simulink model "Power_Model_Official_Pars"  (R2023a)
settings: Solver=ode23t  StartTime=0.0  StopTime=1000  FixedStep=0.01  MaxStep=0.01  RelTol=1e-3  AbsTol=1e-3
values from neighbouring files (symbols this model uses):
  anode_tube_D = 0.01    [fuel_cell_battery_par.mat]
  cathode_tube_D = 0.05    [fuel_cell_battery_par.mat]
  comp_rpm_TLU = [0 1800 3600]    [fuel_cell_battery_par.mat]
  coolant_num_layers = 20    [fuel_cell_battery_par.mat]
  coolant_num_passes = 12    [fuel_cell_battery_par.mat]
  coolant_tube_D = 0.05    [fuel_cell_battery_par.mat]
  coolant_w_channels = 1    [fuel_cell_battery_par.mat]
  env_p = 0.101325    [fuel_cell_battery_par.mat]
  env_T = 20    [fuel_cell_battery_par.mat]
  env_yH20 = 0.0115436377169    [fuel_cell_battery_par.mat]
  env_yO2 = 0.21    [fuel_cell_battery_par.mat]
  radiator_air_area_fins = 11.5625    [fuel_cell_battery_par.mat]
  radiator_air_area_primary = 1.223125    [fuel_cell_battery_par.mat]
  radiator_eta_fin = 0.7    [fuel_cell_battery_par.mat]
  radiator_N_tubes = 25    [fuel_cell_battery_par.mat]
  radiator_rho = 2700    [fuel_cell_battery_par.mat]
  radiator_t_wall = 0.0001    [fuel_cell_battery_par.mat]
  radiator_tube_H = 0.0015    [fuel_cell_battery_par.mat]
  radiator_W = 0.025    [fuel_cell_battery_par.mat]
  stack_area = 280    [fuel_cell_battery_par.mat]
  stack_iL = 1.4    [fuel_cell_battery_par.mat]
  stack_mea_rho = 1800    [fuel_cell_battery_par.mat]
  stack_num_cells = 400    [fuel_cell_battery_par.mat]
  stack_num_channels = 8    [fuel_cell_battery_par.mat]
  stack_t_gdl = 250    [fuel_cell_battery_par.mat]
  stack_t_membrane = 125    [fuel_cell_battery_par.mat]
  stack_w_channels = 1    [fuel_cell_battery_par.mat]
undefined symbols (not defined in the file or in its folder): Bat, f_fc_auxpower, f_fc_currcmd_bpt, f_fc_h2flow, f_fc_heatflow, f_fc_tmpcmd_bpt, f_fc_voltage, Mot, N2_T
libraries: fl_lib x170, nesl_utility x78, FuelCell_lib x32, simulink x5, slpidlib x4, ee_lib x3, autolibshared x1, batteryecm_lib x1, simulink_extras x1
(part 5 of 9)

== system Power_Model_Official_Pars/氧气供给(压缩机)/压缩机查表 ==
  note: 转速_压力比_流量
  Absolute Reference (MA) : fl_lib/Moist Air/Elements/Absolute Reference (MA)
  Absolute Reference (MA)1 : fl_lib/Moist Air/Elements/Absolute Reference (MA)
  Corrected Flow Table : fl_lib/Physical Signals/Lookup Tables/PS Lookup Table (2D)  x1=comp_p_ratio_TLU Pa/Pa  x2=comp_rpm_TLU rpm  f=comp_mdot_corr_TLU kg/s  interp_method=simscape.enum.interpolation.linear  extrap_method=simscape.enum.extrapolation.nearest
  PS Divide : fl_lib/Physical Signals/Functions/PS Divide
  Pressure & Temperature Sensor (MA) : fl_lib/Moist Air/Sensors/Pressure & Temperature Sensor (MA)  reference=foundation.enum.MeasurementReference.difference  pressure=true  pressure_spec=foundation.enum.PressureMeasementSpec.Absolute  temperature=true
      settings: InternalSimscapePortConfiguration="{\"Bottom\":[{\"id\":\"T\",\"label\":\"T\",\"type\":\"output\"}],\"Left\":[{\"id\":\"A\",\"label\":\"A\",\"type\":\"foundation.moist_air.moist_air\"}],\"Right\":[{\"id\":\"B\",\"label\":\"B\",\"type\":\"foundation.moist_air.moist_air\"},{\"id\":\"P\",\"label\":\"P\",\"type\":\"output\"}],\"Top\":[]}"
  Pressure & Temperature Sensor (MA)1 : fl_lib/Moist Air/Sensors/Pressure & Temperature Sensor (MA)  reference=foundation.enum.MeasurementReference.difference  pressure=true  pressure_spec=foundation.enum.PressureMeasementSpec.Absolute  temperature=true
      settings: InternalSimscapePortConfiguration="{\"Bottom\":[{\"id\":\"T\",\"label\":\"T\",\"type\":\"output\"}],\"Left\":[{\"id\":\"A\",\"label\":\"A\",\"type\":\"foundation.moist_air.moist_air\"}],\"Right\":[{\"id\":\"B\",\"label\":\"B\",\"type\":\"foundation.moist_air.moist_air\"},{\"id\":\"P\",\"label\":\"P\",\"type\":\"output\"}],\"Top\":[]}"
  mdot : PMIOPort  Side=Left
  in : PMIOPort  Port=2  Side=Right
  rpm : PMIOPort  Port=3  Side=Right
  out : PMIOPort  Port=4  Side=Right
  connections:
  Pressure & Temperature Sensor (MA)1/RConn2 -- PS Divide/LConn1
  Absolute Reference (MA)1/LConn1 -- Pressure & Temperature Sensor (MA)1/RConn1
  PS Divide/RConn1 -- Corrected Flow Table/LConn1
  rpm/RConn1 -- Corrected Flow Table/LConn2
  Pressure & Temperature Sensor (MA)/RConn2 -- PS Divide/LConn2
  in/RConn1 -- Pressure & Temperature Sensor (MA)/LConn1
  Absolute Reference (MA)/LConn1 -- Pressure & Temperature Sensor (MA)/RConn1
  Pressure & Temperature Sensor (MA)1/LConn1 -- out/RConn1
  mdot/RConn1 -- Corrected Flow Table/RConn1

== system Power_Model_Official_Pars/阳极加湿器/Proportional Control ==
  RH_set : Inport
  RH_meas : Inport  Port=2
  Gain : Gain  Gain=0.1
  Saturation : Saturate  UpperLimit=inf  LowerLimit=0  ZeroCross=off
  Sum : Sum  Inputs=|+-
  Transfer Fcn : TransferFcn  Denominator=[1 1]
  Mw : Outport
  wires:
  Transfer Fcn/1 -> Mw/1
  Gain/1 -> Saturation/1
  Sum/1 -> Gain/1
  RH_set/1 -> Sum/1
  RH_meas/1 -> Sum/2
  Saturation/1 -> Transfer Fcn/1

== system Power_Model_Official_Pars/阴极加湿器/Proportional Control ==
  RH_set : Inport
  RH_meas : Inport  Port=2
  Gain : Gain  Gain=0.1
  Saturation : Saturate  UpperLimit=inf  LowerLimit=0  ZeroCross=off
  Sum : Sum  Inputs=|+-
  Transfer Fcn : TransferFcn  Denominator=[1 1]
  Mw : Outport
  wires:
  RH_set/1 -> Sum/1
  Sum/1 -> Gain/1
  RH_meas/1 -> Sum/2
  Transfer Fcn/1 -> Mw/1
  Gain/1 -> Saturation/1
  Saturation/1 -> Transfer Fcn/1

== system Power_Model_Official_Pars/阴极排放/Pressure Relief Valve ==
  note: 实际输出压力
  note: 设定输出压力
  Absolute Reference (MA) : fl_lib/Moist Air/Elements/Absolute Reference (MA)
  PS Add : fl_lib/Physical Signals/Functions/PS Add
  PS Constant : fl_lib/Physical Signals/Sources/PS Constant  constant=r_min^2
  PS Gain : fl_lib/Physical Signals/Functions/PS Gain  gain=(r_max^2 - r_min^2)/p_range 1/MPa
  PS Gain1 : fl_lib/Physical Signals/Functions/PS Gain  gain=pi*D^2/4 m^2
  PS Subtract : fl_lib/Physical Signals/Functions/PS Subtract
  Pressure & Temperature Sensor (MA) : fl_lib/Moist Air/Sensors/Pressure & Temperature Sensor (MA)  reference=foundation.enum.MeasurementReference.difference  pressure=true  pressure_spec=foundation.enum.PressureMeasementSpec.Absolute  temperature=true
      settings: InternalSimscapePortConfiguration="{\"Bottom\":[{\"id\":\"T\",\"label\":\"T\",\"type\":\"output\"}],\"Left\":[{\"id\":\"A\",\"label\":\"A\",\"type\":\"foundation.moist_air.moist_air\"}],\"Right\":[{\"id\":\"B\",\"label\":\"B\",\"type\":\"foundation.moist_air.moist_air\"},{\"id\":\"P\",\"label\":\"P\",\"type\":\"output\"}],\"Top\":[]}"
  Valve : fl_lib/Moist Air/Elements/Local Restriction (MA)  restriction_type=foundation.enum.restriction_type.variable  restriction_area=0.001 m^2  min_area=pi*(r_min*D)^2/4 m^2  max_area=pi*(r_max*D)^2/4 m^2  area=pi*D^2/4 m^2  Cd=0.64  B_lam=0.999
  A : PMIOPort  Side=Left
  B : PMIOPort  Port=2  Side=Right
  p_set : PMIOPort  Port=3  Side=Left
  connections:
  p_set/RConn1 -- PS Subtract/LConn2
  Pressure & Temperature Sensor (MA)/RConn2 -- PS Subtract/LConn1
  PS Add/LConn2 -- PS Constant/RConn1
  PS Gain/RConn1 -- PS Add/LConn1
  Pressure & Temperature Sensor (MA)/LConn1 -- A/RConn1 -- Valve/LConn1
  Valve/RConn1 -- B/RConn1
  Absolute Reference (MA)/LConn1 -- Pressure & Temperature Sensor (MA)/RConn1
  PS Gain1/RConn1 -- Valve/LConn2
  PS Gain/LConn1 -- PS Subtract/RConn1
  PS Add/RConn1 -- PS Gain1/LConn1

== system Power_Model_Official_Pars/Electrical Load/Inputs/Drive Cycle Power Demand ==
  From Workspace : FromWorkspace  VariableName=[drive_cycle_time, drive_cycle_power]
  PS Divide : fl_lib/Physical Signals/Functions/PS Divide
  PS-Simulink Converter : nesl_utility/PS-Simulink Converter  PhysicalDomain=network_engine_domain  SubClassName=ps_output  LeftPortType=input  RightPortType=output  PseudoPeriodic=off  Frequencies=[]  VectorFormat=1-D array  Unit=V  AffineConversion=off
  PS-Simulink Converter1 : nesl_utility/PS-Simulink Converter  PhysicalDomain=network_engine_domain  SubClassName=ps_output  LeftPortType=input  RightPortType=output  PseudoPeriodic=off  Frequencies=[]  VectorFormat=1-D array  Unit=A  AffineConversion=off
  Simulink-PS Converter : nesl_utility/Simulink-PS Converter  PhysicalDomain=network_engine_domain  SubClassName=ps_input  LeftPortType=input  RightPortType=output  PseudoPeriodic=off  Frequencies=[]  NoiseDistribution=none  NoiseParameters=[]  Unit=kW  AffineConversion=off  FilteringAndDerivatives=provide  SimscapeFilterOrder=1  InputFilterTimeConstant=0.001  UdotUserProvided=0
  i : PMIOPort  Side=Left
  v : PMIOPort  Port=2  Side=Left
  tag scope: i_stack=global, v_stack=global
  wires:
  From Workspace/1 -> Simulink-PS Converter/1
  PS-Simulink Converter/1 -> [v_stack]
  PS-Simulink Converter1/1 -> [i_stack]
  connections:
  PS Divide/LConn1 -- Simulink-PS Converter/RConn1
  i/RConn1 -- PS Divide/RConn1 -- PS-Simulink Converter1/LConn1
  v/RConn1 -- PS-Simulink Converter/LConn1 -- PS Divide/LConn2

== system Power_Model_Official_Pars/Electrical Load/Inputs/Ramp Current Demand ==
  PS-Simulink Converter : nesl_utility/PS-Simulink Converter  PhysicalDomain=network_engine_domain  SubClassName=ps_output  LeftPortType=input  RightPortType=output  PseudoPeriodic=off  Frequencies=[]  VectorFormat=1-D array  Unit=V  AffineConversion=off
  Ramp : simulink/Sources/Ramp  slope=stack_iL * stack_area /1000  start=0  InitialOutput=1e-6 * stack_iL * stack_area
  Simulink-PS Converter : nesl_utility/Simulink-PS Converter  PhysicalDomain=network_engine_domain  SubClassName=ps_input  LeftPortType=input  RightPortType=output  PseudoPeriodic=off  Frequencies=[]  NoiseDistribution=none  NoiseParameters=[]  Unit=A  AffineConversion=off  FilteringAndDerivatives=provide  SimscapeFilterOrder=1  InputFilterTimeConstant=0.001  UdotUserProvided=0
  i : PMIOPort  Side=Left
  v : PMIOPort  Port=2  Side=Left
  tag scope: i_stack=global, v_stack=global
  wires:
  Ramp/1 -> Simulink-PS Converter/1, [i_stack]
  PS-Simulink Converter/1 -> [v_stack]
  connections:
  Simulink-PS Converter/RConn1 -- i/RConn1
  v/RConn1 -- PS-Simulink Converter/LConn1

== system Power_Model_Official_Pars/Electrical Load/Inputs/Step Current Demand ==
  PS-Simulink Converter : nesl_utility/PS-Simulink Converter  PhysicalDomain=network_engine_domain  SubClassName=ps_output  LeftPortType=input  RightPortType=output  PseudoPeriodic=off  Frequencies=[]  VectorFormat=1-D array  Unit=V  AffineConversion=off
  Simulink-PS Converter : nesl_utility/Simulink-PS Converter  PhysicalDomain=network_engine_domain  SubClassName=ps_input  LeftPortType=input  RightPortType=output  PseudoPeriodic=off  Frequencies=[]  NoiseDistribution=none  NoiseParameters=[]  Unit=A  AffineConversion=off  FilteringAndDerivatives=provide  SimscapeFilterOrder=1  InputFilterTimeConstant=0.001  UdotUserProvided=0
  Step : Step  Time=0  Before=1e-6 * stack_iL * stack_area  After=stack_iL * stack_area  SampleTime=0
  i : PMIOPort  Side=Left
  v : PMIOPort  Port=2  Side=Left
  tag scope: i_stack=global, v_stack=global
  wires:
  Step/1 -> [i_stack], Simulink-PS Converter/1
  PS-Simulink Converter/1 -> [v_stack]
  connections:
  Simulink-PS Converter/RConn1 -- i/RConn1
  PS-Simulink Converter/LConn1 -- v/RConn1

== system Power_Model_Official_Pars/Electrical Load1/Inputs/Drive Cycle Power Demand ==
  From Workspace : FromWorkspace  VariableName=[drive_cycle_time, drive_cycle_power]
  PS Divide : fl_lib/Physical Signals/Functions/PS Divide
  PS-Simulink Converter : nesl_utility/PS-Simulink Converter  PhysicalDomain=network_engine_domain  SubClassName=ps_output  LeftPortType=input  RightPortType=output  PseudoPeriodic=off  Frequencies=[]  VectorFormat=1-D array  Unit=V  AffineConversion=off
  PS-Simulink Converter1 : nesl_utility/PS-Simulink Converter  PhysicalDomain=network_engine_domain  SubClassName=ps_output  LeftPortType=input  RightPortType=output  PseudoPeriodic=off  Frequencies=[]  VectorFormat=1-D array  Unit=A  AffineConversion=off
  Simulink-PS Converter : nesl_utility/Simulink-PS Converter  PhysicalDomain=network_engine_domain  SubClassName=ps_input  LeftPortType=input  RightPortType=output  PseudoPeriodic=off  Frequencies=[]  NoiseDistribution=none  NoiseParameters=[]  Unit=kW  AffineConversion=off  FilteringAndDerivatives=provide  SimscapeFilterOrder=1  InputFilterTimeConstant=0.001  UdotUserProvided=0
  i : PMIOPort  Side=Left
  v : PMIOPort  Port=2  Side=Left
  tag scope: i_stack=global, v_stack=global
  wires:
  From Workspace/1 -> Simulink-PS Converter/1
  PS-Simulink Converter/1 -> [v_stack]
  PS-Simulink Converter1/1 -> [i_stack]
  connections:
  PS Divide/LConn1 -- Simulink-PS Converter/RConn1
  i/RConn1 -- PS Divide/RConn1 -- PS-Simulink Converter1/LConn1
  v/RConn1 -- PS-Simulink Converter/LConn1 -- PS Divide/LConn2

== system Power_Model_Official_Pars/Electrical Load1/Inputs/Ramp Current Demand ==
  PS-Simulink Converter : nesl_utility/PS-Simulink Converter  PhysicalDomain=network_engine_domain  SubClassName=ps_output  LeftPortType=input  RightPortType=output  PseudoPeriodic=off  Frequencies=[]  VectorFormat=1-D array  Unit=V  AffineConversion=off
  Ramp : simulink/Sources/Ramp  slope=stack_iL * stack_area /1000  start=0  InitialOutput=1e-6 * stack_iL * stack_area
  Simulink-PS Converter : nesl_utility/Simulink-PS Converter  PhysicalDomain=network_engine_domain  SubClassName=ps_input  LeftPortType=input  RightPortType=output  PseudoPeriodic=off  Frequencies=[]  NoiseDistribution=none  NoiseParameters=[]  Unit=A  AffineConversion=off  FilteringAndDerivatives=provide  SimscapeFilterOrder=1  InputFilterTimeConstant=0.001  UdotUserProvided=0
  i : PMIOPort  Side=Left
  v : PMIOPort  Port=2  Side=Left
  tag scope: i_stack=global, v_stack=global
  wires:
  Ramp/1 -> Simulink-PS Converter/1, [i_stack]
  PS-Simulink Converter/1 -> [v_stack]
  connections:
  Simulink-PS Converter/RConn1 -- i/RConn1
  v/RConn1 -- PS-Simulink Converter/LConn1

== system Power_Model_Official_Pars/Electrical Load1/Inputs/Step Current Demand ==
  PS-Simulink Converter : nesl_utility/PS-Simulink Converter  PhysicalDomain=network_engine_domain  SubClassName=ps_output  LeftPortType=input  RightPortType=output  PseudoPeriodic=off  Frequencies=[]  VectorFormat=1-D array  Unit=V  AffineConversion=off
  Simulink-PS Converter : nesl_utility/Simulink-PS Converter  PhysicalDomain=network_engine_domain  SubClassName=ps_input  LeftPortType=input  RightPortType=output  PseudoPeriodic=off  Frequencies=[]  NoiseDistribution=none  NoiseParameters=[]  Unit=A  AffineConversion=off  FilteringAndDerivatives=provide  SimscapeFilterOrder=1  InputFilterTimeConstant=0.001  UdotUserProvided=0
  Step : Step  Time=0  Before=1e-6 * stack_iL * stack_area  After=stack_iL * stack_area  SampleTime=0
  i : PMIOPort  Side=Left
  v : PMIOPort  Port=2  Side=Left
  tag scope: i_stack=global, v_stack=global
  wires:
  Step/1 -> [i_stack], Simulink-PS Converter/1
  PS-Simulink Converter/1 -> [v_stack]
  connections:
  Simulink-PS Converter/RConn1 -- i/RConn1
  PS-Simulink Converter/LConn1 -- v/RConn1

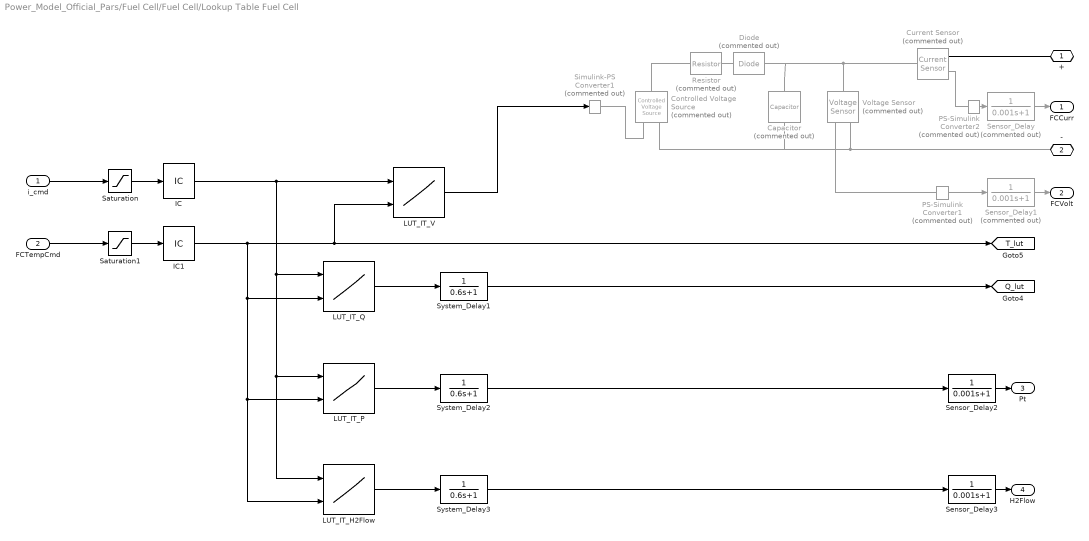
== system Power_Model_Official_Pars/Fuel Cell/Fuel Cell/Lookup Table Fuel Cell ==
  i_cmd : Inport
  FCTempCmd : Inport  Port=2
  Capacitor : fl_lib/Electrical/Electrical Elements/Capacitor  Commented=on  c=1e-6 F  r=1e-6 Ohm  g=0 1/Ohm  i_specify=off  i_priority=None  i=0 A  i_nominal_specify=off  i_nominal_unit=A  i_nominal_value=1  v_specify=off  v_priority=None  v=0 V  v_nominal_specify=off  v_nominal_unit=V  v_nominal_value=1  vc_specify=on  vc_priority=High  vc=f_fc_voltage(1) V  vc_nominal_specify=off  vc_nominal_unit=V  vc_nominal_value=1
  Controlled Voltage Source : fl_lib/Electrical/Electrical Sources/Controlled Voltage Source  Commented=on
  Current Sensor : fl_lib/Electrical/Electrical Sensors/Current Sensor  Commented=on
  Diode : fl_lib/Electrical/Electrical Elements/Diode  Commented=on  Vf=0.6 V  Ron=0.3 Ohm  Goff=1e-8 1/Ohm  i_specify=off  i_priority=None  i=0 A  i_nominal_specify=off  i_nominal_unit=A  i_nominal_value=1  v_specify=off  v_priority=None  v=0 V  v_nominal_specify=off  v_nominal_unit=V  v_nominal_value=1
  IC : InitialCondition  Value=f_fc_currcmd_bpt(1)
  IC1 : InitialCondition  Value=f_fc_tmpcmd_bpt(1)
  LUT_IT_H2Flow : Lookup_n-D  BreakpointsForDimension1=f_fc_currcmd_bpt  BreakpointsForDimension2=f_fc_tmpcmd_bpt  Table=f_fc_h2flow  InternalRulePriority=Speed  RndMeth=Simplest
      settings: InputPortMap=u0,u1
  LUT_IT_P : Lookup_n-D  BreakpointsForDimension1=f_fc_currcmd_bpt  BreakpointsForDimension2=f_fc_tmpcmd_bpt  Table=f_fc_auxpower  InternalRulePriority=Speed  RndMeth=Simplest
      settings: InputPortMap=u0,u1
  LUT_IT_Q : Lookup_n-D  BreakpointsForDimension1=f_fc_currcmd_bpt  BreakpointsForDimension2=f_fc_tmpcmd_bpt  Table=f_fc_heatflow  InternalRulePriority=Speed  RndMeth=Simplest
      settings: InputPortMap=u0,u1
  LUT_IT_V : Lookup_n-D  BreakpointsForDimension1=f_fc_currcmd_bpt  BreakpointsForDimension2=f_fc_tmpcmd_bpt  Table=f_fc_voltage  InternalRulePriority=Speed  RndMeth=Simplest
      settings: InputPortMap=u0,u1
  PS-Simulink Converter1 : nesl_utility/PS-Simulink Converter  Commented=on  PhysicalDomain=network_engine_domain  SubClassName=ps_output  LeftPortType=input  RightPortType=output  PseudoPeriodic=off  Frequencies=[]  VectorFormat=1-D array  Unit=inherit  AffineConversion=off
  PS-Simulink Converter2 : nesl_utility/PS-Simulink Converter  Commented=on  PhysicalDomain=network_engine_domain  SubClassName=ps_output  LeftPortType=input  RightPortType=output  PseudoPeriodic=off  Frequencies=[]  VectorFormat=1-D array  Unit=1  AffineConversion=off
  Resistor : fl_lib/Electrical/Electrical Elements/Resistor  Commented=on  R=1e-3 Ohm  i_specify=off  i_priority=None  i=0 A  i_nominal_specify=off  i_nominal_unit=A  i_nominal_value=1  v_specify=off  v_priority=None  v=0 V  v_nominal_specify=off  v_nominal_unit=V  v_nominal_value=1
  Saturation : Saturate  UpperLimit=max(f_fc_currcmd_bpt)  LowerLimit=0
  Saturation1 : Saturate  UpperLimit=max(f_fc_tmpcmd_bpt)  LowerLimit=0
  Sensor_Delay : TransferFcn  Commented=on  Denominator=[0.001 1]
  Sensor_Delay1 : TransferFcn  Commented=on  Denominator=[0.001 1]
  Sensor_Delay2 : TransferFcn  Denominator=[0.001 1]
  Sensor_Delay3 : TransferFcn  Denominator=[0.001 1]
  Simulink-PS Converter1 : nesl_utility/Simulink-PS Converter  Commented=on  PhysicalDomain=network_engine_domain  SubClassName=ps_input  LeftPortType=input  RightPortType=output  PseudoPeriodic=off  Frequencies=[]  NoiseDistribution=none  NoiseParameters=[]  Unit=V  AffineConversion=off  FilteringAndDerivatives=provide  SimscapeFilterOrder=1  InputFilterTimeConstant=0.001  UdotUserProvided=0
  System_Delay1 : TransferFcn  Denominator=[0.6 1]
  System_Delay2 : TransferFcn  Denominator=[0.6 1]
  System_Delay3 : TransferFcn  Denominator=[0.6 1]
  Voltage Sensor : fl_lib/Electrical/Electrical Sensors/Voltage Sensor  Commented=on
  + : PMIOPort  Side=Right
  - : PMIOPort  Port=2  Side=Right
  FCCurr : Outport
  FCVolt : Outport  Port=2
  Pt : Outport  Port=3
  H2Flow : Outport  Port=4
  tag scope: Q_lut=global, T_lut=global
  wires:
  PS-Simulink Converter2/1 -> Sensor_Delay/1
  PS-Simulink Converter1/1 -> Sensor_Delay1/1
  Sensor_Delay/1 -> FCCurr/1
  Sensor_Delay1/1 -> FCVolt/1
  System_Delay2/1 -> Sensor_Delay2/1
  Sensor_Delay2/1 -> Pt/1
  Sensor_Delay3/1 -> H2Flow/1
  System_Delay3/1 -> Sensor_Delay3/1
  Saturation/1 -> IC/1
  Saturation1/1 -> IC1/1
  i_cmd/1 -> Saturation/1
  FCTempCmd/1 -> Saturation1/1
  LUT_IT_H2Flow/1 -> System_Delay3/1
  LUT_IT_P/1 -> System_Delay2/1
  IC1/1 -> LUT_IT_V/2, [T_lut], LUT_IT_H2Flow/2, LUT_IT_P/2, LUT_IT_Q/2
  IC/1 -> LUT_IT_H2Flow/1, LUT_IT_P/1, LUT_IT_Q/1, LUT_IT_V/1
  LUT_IT_Q/1 -> System_Delay1/1
  System_Delay1/1 -> [Q_lut]
  LUT_IT_V/1 -> Simulink-PS Converter1/1
  connections:
  Voltage Sensor/LConn1 -- Current Sensor/LConn1 -- Diode/RConn1 -- Capacitor/LConn1
  Simulink-PS Converter1/RConn1 -- Controlled Voltage Source/RConn1
  PS-Simulink Converter2/LConn1 -- Current Sensor/RConn1
  +/RConn1 -- Current Sensor/RConn2
  Voltage Sensor/RConn2 -- -/RConn1 -- Controlled Voltage Source/RConn2 -- Capacitor/RConn1
  PS-Simulink Converter1/LConn1 -- Voltage Sensor/RConn1
  Resistor/RConn1 -- Diode/LConn1
  Resistor/LConn1 -- Controlled Voltage Source/LConn1
